simulink model "UAV_USV_Simulator"  (R2017b)
settings: Solver=ode3  StartTime=0.0  StopTime=15  FixedStep=0.01  RelTol=1e-3
PreLoadFcn:
  | addpath(genpath(fileparts(which (bdroot))))
  | 
  | CascadedPID=Simulink.Variant('ControlType==0');
  | InverseKin=Simulink.Variant('ControlType==1');
  | 
  | ControlType = 0;
  | Waypoints = [10 10 ; -10 10 ; -10 -10; 10 -10; 0 0 ];
  | WaypointsX = Waypoints(:,1)'/3;
  | WaypointsY = Waypoints(:,2)'/3;
  | StriderSpeedCmd = 0;
  | 
  | ax=0;
  | ay=0;
  | LandingSchedule = 5;
  | EnableVTOL=1;
  | Psi_cmd = 0;
  | Alt_cmd = 1;
  | 
  | AccRadius =0.5;
  | AppAlt =1;
  | e = 0.1;
PostLoadFcn:
  | addpath(genpath(fileparts(which (bdroot))))
model workspace (MAT data in the model file):
  MCOS : class17 (value not decoded)
  MCOS : class17 (value not decoded)
  MCOS : class17 (value not decoded)
  MCOS : class17 (value not decoded)
  MCOS : class17 (value not decoded)
  MCOS : class17 (value not decoded)
undefined symbols (not defined in the file or in its folder): magnitude, sigbuilder_block
libraries: simulink x12, simulink_extras x12, vrlib x5, dsparch4 x1, sharedtransform x1, dspswit3 x1
(part 2 of 2)

== system UAV_USV_Simulator/Attitude Controller/Altitude Control/Altitude controller/Inverse Kinematics Altitude ==
  Alt_cmd : Inport
  Bus Selector1 : BusSelector  OutputSignals=Alt_cmd
  Gain1 : Gain  Gain=1/(4*CT)
  Gain2 : Gain  Gain=100*60/(MaxRPM*2*pi)
  Sqrt : Sqrt  SaturateOnIntegerOverflow=on
  Out : Outport
  wires:
  Gain2/1 -> Out/1
  Sqrt/1 -> Gain2/1
  Alt_cmd/1 -> Bus Selector1/1
  Bus Selector1/1 -> Gain1/1  "<Alt_cmd>"
  Gain1/1 -> Sqrt/1

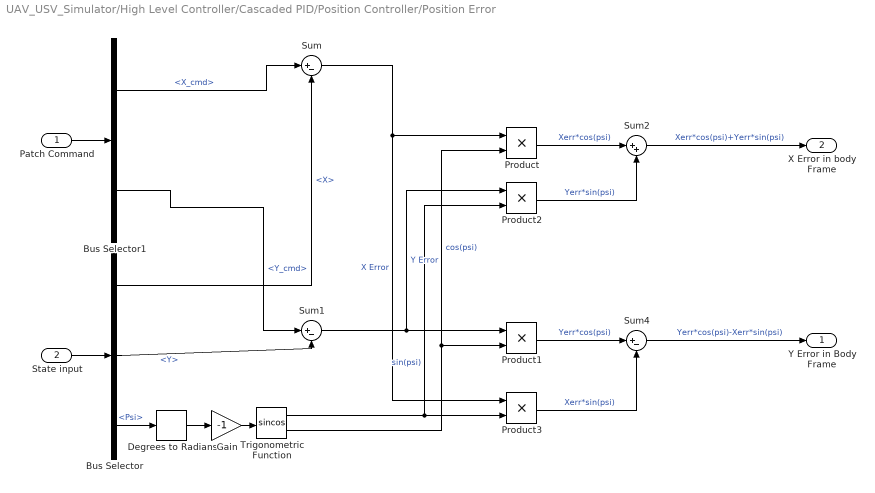
== system UAV_USV_Simulator/High Level Controller/Cascaded PID/Position Controller/Position Error ==
  Patch Command : Inport
  State input : Inport  Port=2
  Bus Selector : BusSelector  OutputSignals=X,Y,Psi
  Bus Selector1 : BusSelector  OutputSignals=X_cmd,Y_cmd
  Degrees to Radians : simulink_extras/Transformations/Degrees to Radians
  Gain : Gain  Gain=-1
  Product{,1..3} (4 alike) : Product
  Sum : Sum  Inputs=|+-
  Sum1 : Sum  Inputs=|+-
  Sum2 : Sum  Inputs=|++
  Sum4 : Sum  Inputs=|+-
  Trigonometric Function : Trigonometry  Operator=sincos
  Y Error in Body Frame : Outport
  X Error in body Frame : Outport  Port=2
  wires:
  State input/1 -> Bus Selector/1
  Patch Command/1 -> Bus Selector1/1
  Bus Selector/2 -> Sum1/2  "<Y>"
  Bus Selector/1 -> Sum/2  "<X>"
  Bus Selector1/1 -> Sum/1  "<X_cmd>"
  Bus Selector1/2 -> Sum1/1  "<Y_cmd>"
  Bus Selector/3 -> Degrees to Radians/1  "<Psi>"
  Degrees to Radians/1 -> Gain/1
  Sum4/1 -> Y Error in Body Frame/1  "Yerr*cos(psi)-Xerr*sin(psi)"
  Product3/1 -> Sum4/2  "Xerr*sin(psi)"
  Sum1/1 -> Product1/1, Product2/1  "Y Error"
  Trigonometric Function/1 -> Product3/2, Product2/2  "sin(psi)"
  Sum2/1 -> X Error in body Frame/1  "Xerr*cos(psi)+Yerr*sin(psi)"
  Sum/1 -> Product/1, Product3/1  "X Error"
  Trigonometric Function/2 -> Product1/2, Product/2  "cos(psi)"
  Product/1 -> Sum2/1  "Xerr*cos(psi)"
  Product2/1 -> Sum2/2  "Yerr*sin(psi)"
  Product1/1 -> Sum4/1  "Yerr*cos(psi)"
  Gain/1 -> Trigonometric Function/1

== system UAV_USV_Simulator/High Level Controller/Cascaded PID/Velocity Controller/Phi Command Control ==
  Desired Yb Velocity : Inport
  Yb Velocity : Inport  Port=2
  Bus Selector : BusSelector  OutputSignals=V
  Gain : Gain  Gain=-1
  PID Controller4 : simulink/Continuous/PID Controller  Controller=PID  TimeDomain=Continuous-time  SampleTime=-1  IntegratorMethod=Forward Euler  FilterMethod=Forward Euler  Form=Parallel  UseFilter=on  ControllerParametersSource=internal  P=19.6600401691244  I=0  D=0.259478709550943  N=3.0476144677615  InitialConditionSource=internal  InitialConditionForIntegrator=0  InitialConditionForFilter=0  ExternalReset=none  LimitOutput=on  UpperSaturationLimit=15  LowerSaturationLimit=-15  LinearizeAsGain=on  AntiWindupMode=none  Kb=1  TrackingMode=off  Kt=1  PParamMin=[]  PParamMax=[]  IParamMin=[]  IParamMax=[]  DParamMin=[]  DParamMax=[]  NParamMin=[]  NParamMax=[]  KbParamMin=[]  KbParamMax=[]  KtParamMin=[]  KtParamMax=[]  POutMin=[]  POutMax=[]  IOutMin=[]  IOutMax=[]  DOutMin=[]  DOutMax=[]  NOutMin=[]  NOutMax=[]  KbOutMin=[]  KbOutMax=[]  KtOutMin=[]  KtOutMax=[]  IntegratorOutMin=[]  IntegratorOutMax=[]  FilterOutMin=[]  FilterOutMax=[]  SumOutMin=[]  SumOutMax=[]  SumI1OutMin=[]  SumI1OutMax=[]  SumI2OutMin=[]  SumI2OutMax=[]  SumI3OutMin=[]  SumI3OutMax=[]  SumDOutMin=[]  SumDOutMax=[]  SaturationOutMin=[]  SaturationOutMax=[]  IntegratorContinuousStateAttributes=''  IntegratorStateMustResolveToSignalObject=off  IntegratorRTWStateStorageClass=Auto  FilterContinuousStateAttributes=''  FilterStateMustResolveToSignalObject=off  FilterRTWStateStorageClass=Auto  DifferentiatorICPrevScaledInput=0  DifferentiatorOutMin=[]  DifferentiatorOutMax=[]  InitialConditionSetting=State (most efficient)  FilterDiffOutCoefMin=[]  FilterDiffOutCoefMax=[]  SumDenOutMin=[]  SumDenOutMax=[]  SumNumOutMin=[]  SumNumOutMax=[]  ReciprocalOutMin=[]  ReciprocalOutMax=[]  DivideOutMin=[]  DivideOutMax=[]  TunerSelectOption=Transfer Function Based (PID Tuner App)
  Sum3 : Sum  Inputs=|+-
  Phi_cmd : Outport
  wires:
  PID Controller4/1 -> Gain/1  "Phi_cmd"
  Sum3/1 -> PID Controller4/1  "Velocity Error"
  Desired Yb Velocity/1 -> Sum3/1
  Yb Velocity/1 -> Bus Selector/1
  Gain/1 -> Phi_cmd/1
  Bus Selector/1 -> Sum3/2  "<V>"

== system UAV_USV_Simulator/High Level Controller/Cascaded PID/Velocity Controller/Theta Command Control ==
  Desired Xb Velocity : Inport
  Xb Velocity : Inport  Port=2
  Bus Selector : BusSelector  OutputSignals=U
  Gain : Gain  Gain=-1
  PID Controller4 : simulink/Continuous/PID Controller  Controller=PID  TimeDomain=Continuous-time  SampleTime=-1  IntegratorMethod=Forward Euler  FilterMethod=Forward Euler  Form=Parallel  UseFilter=on  ControllerParametersSource=internal  P=19.6600401691244  I=0  D=0.259478709550943  N=3.0476144677615  InitialConditionSource=internal  InitialConditionForIntegrator=0  InitialConditionForFilter=0  ExternalReset=none  LimitOutput=on  UpperSaturationLimit=15  LowerSaturationLimit=-15  LinearizeAsGain=on  AntiWindupMode=none  Kb=1  TrackingMode=off  Kt=1  PParamMin=[]  PParamMax=[]  IParamMin=[]  IParamMax=[]  DParamMin=[]  DParamMax=[]  NParamMin=[]  NParamMax=[]  KbParamMin=[]  KbParamMax=[]  KtParamMin=[]  KtParamMax=[]  POutMin=[]  POutMax=[]  IOutMin=[]  IOutMax=[]  DOutMin=[]  DOutMax=[]  NOutMin=[]  NOutMax=[]  KbOutMin=[]  KbOutMax=[]  KtOutMin=[]  KtOutMax=[]  IntegratorOutMin=[]  IntegratorOutMax=[]  FilterOutMin=[]  FilterOutMax=[]  SumOutMin=[]  SumOutMax=[]  SumI1OutMin=[]  SumI1OutMax=[]  SumI2OutMin=[]  SumI2OutMax=[]  SumI3OutMin=[]  SumI3OutMax=[]  SumDOutMin=[]  SumDOutMax=[]  SaturationOutMin=[]  SaturationOutMax=[]  IntegratorContinuousStateAttributes=''  IntegratorStateMustResolveToSignalObject=off  IntegratorRTWStateStorageClass=Auto  FilterContinuousStateAttributes=''  FilterStateMustResolveToSignalObject=off  FilterRTWStateStorageClass=Auto  DifferentiatorICPrevScaledInput=0  DifferentiatorOutMin=[]  DifferentiatorOutMax=[]  InitialConditionSetting=State (most efficient)  FilterDiffOutCoefMin=[]  FilterDiffOutCoefMax=[]  SumDenOutMin=[]  SumDenOutMax=[]  SumNumOutMin=[]  SumNumOutMax=[]  ReciprocalOutMin=[]  ReciprocalOutMax=[]  DivideOutMin=[]  DivideOutMax=[]  TunerSelectOption=Transfer Function Based (PID Tuner App)
  Sum3 : Sum  Inputs=|+-
  The_cmd : Outport
  wires:
  Xb Velocity/1 -> Bus Selector/1
  Sum3/1 -> PID Controller4/1  "Velocity Error"
  Desired Xb Velocity/1 -> Sum3/1
  PID Controller4/1 -> Gain/1  "Theta comand"
  Bus Selector/1 -> Sum3/2  "<U>"
  Gain/1 -> The_cmd/1

== system UAV_USV_Simulator/High Level Controller/Inverse kinematics architecture/Thrust and angle calculation3/Norm calculation ==
  Thrust value : Inport
  Math Function : Math  Operator=square  SaturateOnIntegerOverflow=on
  Math Function1 : Math  Operator=sqrt  SaturateOnIntegerOverflow=on
  Scope : Scope  NumInputPorts=4
  Sum of Elements : Sum  Inputs=+
  Thrust value1 : Outport
  wires:
  Thrust value/1 -> Scope/1, Math Function/1
  Math Function1/1 -> Scope/4, Thrust value1/1  "Thrust value"
  Math Function/1 -> Scope/2, Sum of Elements/1
  Sum of Elements/1 -> Scope/3, Math Function1/1

== system UAV_USV_Simulator/High Level Controller/Inverse kinematics architecture/Thrust and angle calculation3/Subsystem ==
  In1 : Inport
  Psi_cmd : Inport  Port=2
  Cross Product : vrlib/Utilities/Cross Product
      settings: SourceProductBaseCode=VR
  Cross Product1 : vrlib/Utilities/Cross Product
      settings: SourceProductBaseCode=VR
  Normalize Vector : vrlib/Utilities/Normalize Vector  maxzero=0
      settings: SourceProductName=Simulink 3D Animation  SourceProductBaseCode=VR
  Normalize Vector1 : vrlib/Utilities/Normalize Vector  maxzero=0
      settings: SourceProductName=Simulink 3D Animation  SourceProductBaseCode=VR
  Normalize Vector2 : vrlib/Utilities/Normalize Vector  maxzero=0
      settings: SourceProductName=Simulink 3D Animation  SourceProductBaseCode=VR
  Reshape : Reshape  OutputDimensionality=Column vector (2-D)
  x_c calc : Subsystem
  x_b : Outport
  y_b : Outport  Port=2
  z_b : Outport  Port=3
  t : Outport  Port=4
  wires:
  Cross Product/1 -> Normalize Vector1/1
  Cross Product1/1 -> Normalize Vector2/1
  In1/1 -> Reshape/1
  Psi_cmd/1 -> x_c calc/1(Psi_cmd)
  Reshape/1 -> t/1, Normalize Vector/1  "t"
  Normalize Vector/1 -> z_b/1, Cross Product/1  "z_b"
  x_c calc/1(x_c) -> Cross Product1/2, Cross Product/2  "x_c"
  Normalize Vector2/1 -> x_b/1  "x_b"
  Normalize Vector1/1 -> y_b/1, Cross Product1/1  "y_b"

== system UAV_USV_Simulator/High Level Controller/Inverse kinematics architecture/Thrust and angle calculation3/Subsystem/x_c calc ==
  Psi_cmd : Inport
  Cos : Trigonometry  Operator=cos
  Cos1 : Trigonometry
  Degrees to Radians : simulink_extras/Transformations/Degrees to Radians
  Degrees to Radians1 : simulink_extras/Transformations/Degrees to Radians
  Ground : Ground
  Reshape : Reshape  OutputDimensionality=Column vector (2-D)
  Vector Concatenate1 : Concatenate  NumInputs=3
  x_c : Outport
  wires:
  Cos/1 -> Vector Concatenate1/1
  Degrees to Radians/1 -> Cos/1
  Psi_cmd/1 -> Degrees to Radians1/1, Degrees to Radians/1
  Vector Concatenate1/1 -> Reshape/1
  Cos1/1 -> Vector Concatenate1/2
  Degrees to Radians1/1 -> Cos1/1
  Ground/1 -> Vector Concatenate1/3
  Reshape/1 -> x_c/1

== matlab function UAV_USV_Simulator/Strider V1.0 Control System/Error calculation ==
  data: cHeading input; error output; H_cmd input; Head output; Hcmd output
function [error,Head,Hcmd]= e(cHeading,H_cmd)

k = floor(abs(cHeading)/(2*pi));    % periodicity calculation

if cHeading >= 0 
    heading = cHeading-k*2*pi;      % correcting values over 360º
else  
    heading = cHeading+(k+1)*2*pi;  % correcting values below -360º
end

if abs(heading-H_cmd) > pi && heading-H_cmd < 0 % compute the shorter angle
    error = 2*pi+(heading-H_cmd);               % to the desired heading.
elseif heading-H_cmd >= pi && heading-H_cmd >= 0
    error = (heading-H_cmd)-2*pi;
else
    error= heading-H_cmd;
end
Head=heading;
Hcmd=H_cmd;

== matlab function UAV_USV_Simulator/Strider V1.0 Control System/Heading angle computation/Quadrant selection ==
  data: xsign input; y output; ysign input
function y = fcn(xsign,ysign)
if xsign >= 0 && ysign >= 0
    y = 0;
elseif xsign >= 0 && ysign < 0 
    y= 2*pi;
else
    y = pi;
end;
